simulink model "sampleModel1739_2"  (R2023a)
settings: Solver=VariableStepAuto  StartTime=0.0  StopTime=10.0  RelTol=1e-3
libraries: hdlsllib x4, simulink x1
settings Model: Creator=user1  LastModifiedBy=user1

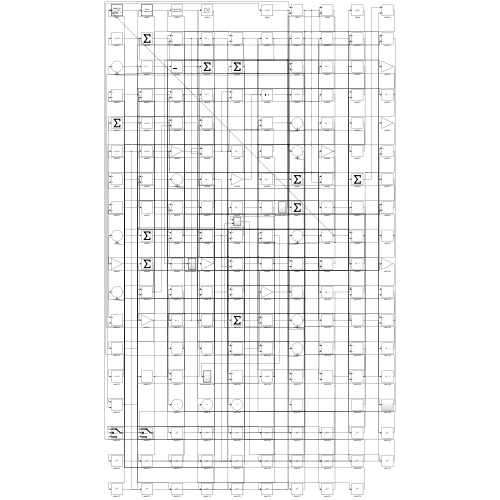
[thumbnail: Simulink's stored preview of the top-level diagram]
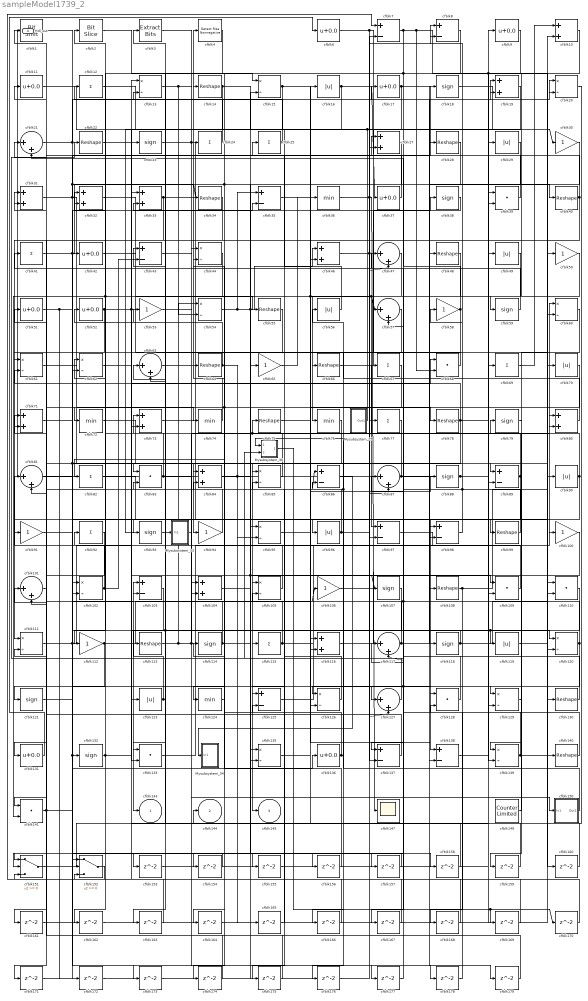
== system sampleModel1739_2 ==
  Mysubsystem_25 : Subsystem  TreatAsAtomicUnit=on  RTWFcnName=Mysubsystem_25
      settings: RTWFcnNameOpts=User specified  RTWFileNameOpts=Use function name
  Mysubsystem_30 : Subsystem  TreatAsAtomicUnit=on  RTWFcnName=Mysubsystem_30
      settings: RTWFcnNameOpts=User specified  RTWFileNameOpts=Use function name
  Mysubsystem_33 : Subsystem  TreatAsAtomicUnit=on  RTWFcnName=Mysubsystem_33
      settings: RTWFcnNameOpts=User specified  RTWFileNameOpts=Use function name
  Mysubsystem_34 : Subsystem  TreatAsAtomicUnit=on  RTWFcnName=Mysubsystem_34
      settings: RTWFcnNameOpts=User specified  RTWFileNameOpts=Use function name
  cfblk1 : hdlsllib/Logic and Bit Operations/Bit Shift  mode=Shift Left Logical  N=0
  cfblk{10,19,27,31..33,46,71,73,80,84,104,116} (13 alike) : Sum  OutDataTypeStr=uint8
  cfblk{30,50,53,58,65,91,94,100,106,112} (10 alike) : Gain  OutDataTypeStr=uint8
  cfblk{21,47,57,63,81,87,101,117,127} (9 alike) : Sum  Inputs=|++  OutDataTypeStr=uint8
  cfblk{13,15,20,44,54,60..62,85,95,102,105,111,120,126,129,135,139} (18 alike) : Product  Inputs=*/  OutDataTypeStr=uint8  RndMeth=Zero  SaturateOnIntegerOverflow=on
  cfblk{7..8,35,43,86,89,97..98,103,125,137..138} (12 alike) : Sum  Inputs=+-  OutDataTypeStr=uint8
  cfblk{18,23,38,59,79,88,93,107,114,118,121,132} (12 alike) : Signum
  cfblk{14,22,28,34,40,48,55,64,66,75,78,99,108,113,130,140} (16 alike) : Reshape
  cfblk{39,68,83,109..110,128,133,141} (8 alike) : DotProduct  OutDataTypeStr=uint8
  cfblk{6,9,11,17,37,42,51..52,131,136} (10 alike) : Bias  Bias=0.0  SaturateOnIntegerOverflow=off
  cfblk{12,24..25,41,67,69,77,82,92,115} (10 alike) : Sum  Inputs=+  OutDataTypeStr=uint8
  cfblk{16,29,49,56,70,90,96,119,123} (9 alike) : Abs  OutDataTypeStr=uint8  SaturateOnIntegerOverflow=off
  cfblk{36,72,74,76,124} (5 alike) : MinMax  OutDataTypeStr=uint8
  cfblk147 : Scope
  cfblk149 : hdlsllib/Sources/Counter Limited  uplimit=7  tsamp=-1
  cfblk150 : Subsystem
      settings: LibrarySourceBlock=|
      | hdlsllib/Ports &
      | Subsystems/Subsystem
  cfblk151 : Switch  OutDataTypeStr=uint8  SaturateOnIntegerOverflow=off  InputSameDT=off
  cfblk152 : Switch  OutDataTypeStr=uint8  SaturateOnIntegerOverflow=off  InputSameDT=off
  cfblk{153..179} (27 alike) : Delay  SampleTime=1
  cfblk2 : hdlsllib/Logic and Bit Operations/Bit Slice  lidx=7  ridx=0
  cfblk3 : simulink/Logic and Bit Operations/Extract Bits  bitsToExtract=Upper half  numBits=8  bitIdxRange=[0 7]  outScalingMode=Preserve fixed-point scaling
      settings: LibrarySourceBlock=|
      | hdlsllib/Logic and Bit
      | Operations/Extract Bits
  cfblk4 : hdlsllib/Logic and Bit Operations/Detect Rise Nonnegative  vinit=0  OutDataTypeStr=uint8
  cfblk143 : Outport  OutDataTypeStr=uint8  VectorParamsAs1DForOutWhenUnconnected=off
  cfblk144 : Outport  Port=2  OutDataTypeStr=uint8  VectorParamsAs1DForOutWhenUnconnected=off
  cfblk145 : Outport  Port=3  OutDataTypeStr=uint8  VectorParamsAs1DForOutWhenUnconnected=off
  Hdl_out : Outport  Port=4  OutDataTypeStr=uint8
  wires:
  cfblk24/1 -> cfblk4/1
  cfblk77/1 -> cfblk94/1
  cfblk34/1 -> cfblk111/1
  cfblk8/1 -> cfblk82/1
  cfblk130/1 -> cfblk92/1
  cfblk85/1 -> cfblk75/1, cfblk43/1
  cfblk140/1 -> cfblk22/1
  cfblk63/1 -> cfblk89/1
  cfblk131/1 -> cfblk6/1
  cfblk65/1 -> cfblk36/1
  cfblk93/1 -> cfblk150/1(In1)
  cfblk79/1 -> cfblk139/1
  cfblk73/1 -> cfblk138/1
  cfblk69/1 -> cfblk10/1
  cfblk36/1 -> cfblk147/1, cfblk138/2
  cfblk21/1 -> cfblk120/1, cfblk17/1
  cfblk33/1 -> cfblk96/1, cfblk102/2
  cfblk66/1 -> cfblk38/1
  cfblk27/1 -> cfblk163/1, cfblk164/1
  cfblk103/1 -> cfblk143/1
  cfblk49/1 -> cfblk97/1, cfblk121/1
  cfblk111/1 -> cfblk23/1, cfblk35/2
  cfblk96/1 -> cfblk71/1, cfblk8/2
  cfblk78/1 -> cfblk145/1, cfblk61/2, cfblk20/2
  cfblk133/1 -> cfblk60/1
  cfblk55/1 -> cfblk61/1
  cfblk108/1 -> cfblk10/2, cfblk168/1
  cfblk70/1 -> cfblk124/1, cfblk101/2
  cfblk31/1 -> cfblk84/1, cfblk27/1
  cfblk37/1 -> cfblk3/1
  cfblk4/1 -> cfblk93/1
  cfblk41/1 -> cfblk140/1, cfblk178/1
  cfblk9/1 -> cfblk72/1, cfblk137/1
  cfblk20/1 -> cfblk144/1
  cfblk115/1 -> cfblk39/1, cfblk21/1
  cfblk151/1 -> cfblk49/1
  cfblk113/1 -> cfblk9/1, cfblk80/1, cfblk54/1
  cfblk87/1 -> cfblk85/1, cfblk179/1
  cfblk106/1 -> cfblk29/1
  cfblk105/1 -> cfblk63/1
  cfblk12/1 -> cfblk98/1
  cfblk47/1 -> cfblk76/1
  cfblk35/1 -> cfblk16/1
  cfblk125/1 -> cfblk50/1
  cfblk141/1 -> cfblk136/1, cfblk31/1
  cfblk124/1 -> cfblk84/2
  cfblk52/1 -> cfblk123/1, cfblk90/1, cfblk81/2
  cfblk123/1 -> cfblk103/1, cfblk153/1
  cfblk71/1 -> cfblk89/2, cfblk156/1
  cfblk116/1 -> cfblk48/1
  cfblk89/1 -> cfblk67/1, cfblk155/1
  cfblk101/1 -> cfblk51/1
  cfblk48/1 -> cfblk115/1
  cfblk6/1 -> cfblk108/1, cfblk127/2
  cfblk149/1 -> cfblk79/1
  cfblk74/1 -> cfblk14/1
  cfblk14/1 -> cfblk63/2, cfblk27/2
  cfblk137/1 -> cfblk101/1
  cfblk17/1 -> cfblk105/1, cfblk40/1
  cfblk2/1 -> cfblk15/1
  cfblk62/1 -> cfblk99/1
  cfblk59/1 -> cfblk47/1
  cfblk15/1 -> cfblk57/1, cfblk78/1, cfblk73/2
  cfblk95/1 -> cfblk88/1
  cfblk138/1 -> cfblk69/1
  cfblk23/1 -> cfblk135/1, cfblk128/1
  cfblk120/1 -> cfblk166/1, cfblk167/1, cfblk64/1
  cfblk42/1 -> cfblk118/1
  cfblk126/1 -> cfblk105/2
  cfblk90/1 -> cfblk151/1, cfblk53/1
  cfblk104/1 -> cfblk65/1
  cfblk29/1 -> cfblk42/1
  cfblk97/1 -> cfblk100/1
  cfblk94/1 -> cfblk13/2
  cfblk150/1(Out1) -> Mysubsystem_30/1(In1), cfblk86/1
  cfblk98/1 -> cfblk58/1
  cfblk54/1 -> cfblk46/1, cfblk126/2, cfblk35/1
  cfblk16/1 -> cfblk37/1, cfblk174/1
  cfblk13/1 -> cfblk44/1, cfblk54/2
  cfblk81/1 -> cfblk98/2
  cfblk92/1 -> cfblk131/1
  cfblk91/1 -> cfblk152/1
  cfblk32/1 -> cfblk55/1
  cfblk114/1 -> cfblk71/2, cfblk28/1
  cfblk10/1 -> cfblk59/1
  cfblk152/1 -> cfblk7/1
  cfblk109/1 -> cfblk2/1
  cfblk83/1 -> cfblk52/1, cfblk80/2
  cfblk56/1 -> cfblk25/1
  cfblk132/1 -> cfblk68/1, cfblk32/2, cfblk162/1
  cfblk11/1 -> cfblk77/1
  cfblk40/1 -> cfblk18/1, cfblk171/1
  cfblk7/1 -> cfblk70/1, cfblk129/2, cfblk68/2, cfblk117/2
  cfblk82/1 -> cfblk110/1
  cfblk110/1 -> cfblk133/1, cfblk133/2, cfblk119/1
  cfblk50/1 -> cfblk112/1, cfblk141/2
  cfblk64/1 -> cfblk32/1, cfblk165/1
  cfblk102/1 -> cfblk81/1, cfblk43/2
  cfblk57/1 -> cfblk83/1
  cfblk75/1 -> cfblk116/2
  cfblk99/1 -> cfblk41/1, cfblk8/1
  cfblk18/1 -> cfblk130/1
  cfblk68/1 -> cfblk66/1
  cfblk60/1 -> cfblk129/1
  cfblk80/1 -> cfblk56/1
  cfblk58/1 -> cfblk126/1, cfblk21/2
  cfblk46/1 -> cfblk47/2, cfblk19/2
  cfblk51/1 -> cfblk132/1, cfblk173/1, cfblk172/1
  cfblk39/1 -> cfblk11/1
  cfblk38/1 -> cfblk33/2
  cfblk139/1 -> cfblk106/1, cfblk73/1, cfblk110/2
  cfblk25/1 -> cfblk12/1, cfblk175/1
  cfblk30/1 -> cfblk135/2
  cfblk72/1 -> cfblk104/1
  cfblk88/1 -> cfblk139/2, Hdl_out/1
  cfblk43/1 -> cfblk104/2
  cfblk44/1 -> cfblk91/1
  cfblk100/1 -> cfblk125/1
  cfblk121/1 -> cfblk103/2
  cfblk117/1 -> cfblk62/1, cfblk20/1
  cfblk61/1 -> cfblk74/1
  cfblk128/1 -> cfblk87/1
  cfblk22/1 -> cfblk109/1
  cfblk112/1 -> cfblk141/1, cfblk46/2
  cfblk1/1 -> cfblk34/1, cfblk127/1
  cfblk3/1 -> cfblk24/1
  cfblk84/1 -> cfblk107/1, cfblk158/1, cfblk95/2
  cfblk118/1 -> cfblk60/2, cfblk113/1
  cfblk136/1 -> cfblk114/1, cfblk86/2
  cfblk135/1 -> cfblk19/1
  cfblk153/1 -> cfblk109/2
  cfblk67/1 -> cfblk154/1
  cfblk154/1 -> cfblk152/2
  cfblk155/1 -> cfblk87/2
  cfblk156/1 -> cfblk44/2
  cfblk28/1 -> cfblk157/1
  cfblk157/1 -> cfblk151/2
  cfblk158/1 -> cfblk83/2
  cfblk129/1 -> cfblk159/1
  cfblk159/1 -> cfblk13/1
  cfblk119/1 -> cfblk160/1
  cfblk160/1 -> cfblk116/1
  cfblk76/1 -> cfblk161/1
  cfblk161/1 -> cfblk39/2
  cfblk162/1 -> cfblk15/2
  cfblk163/1 -> cfblk33/1
  cfblk164/1 -> cfblk120/2
  cfblk165/1 -> cfblk85/2
  cfblk166/1 -> cfblk152/3
  cfblk167/1 -> cfblk125/2
  cfblk168/1 -> cfblk102/1
  cfblk169/1 -> cfblk57/2
  cfblk170/1 -> cfblk151/3
  cfblk171/1 -> cfblk62/2
  cfblk172/1 -> cfblk95/1
  cfblk173/1 -> cfblk7/2
  cfblk174/1 -> cfblk31/2
  cfblk175/1 -> cfblk111/2
  cfblk107/1 -> cfblk176/1
  cfblk176/1 -> cfblk97/2
  cfblk53/1 -> cfblk177/1
  cfblk177/1 -> cfblk117/1
  cfblk178/1 -> cfblk128/2
  cfblk179/1 -> cfblk1/1
  Mysubsystem_25/1(Out1) -> cfblk137/2, cfblk30/1
  Mysubsystem_30/1(Out1) -> cfblk169/1, cfblk170/1
  cfblk127/1 -> Mysubsystem_30/2(In2)
  cfblk19/1 -> Mysubsystem_33/1(In1)
  cfblk86/1 -> Mysubsystem_34/1(In1)

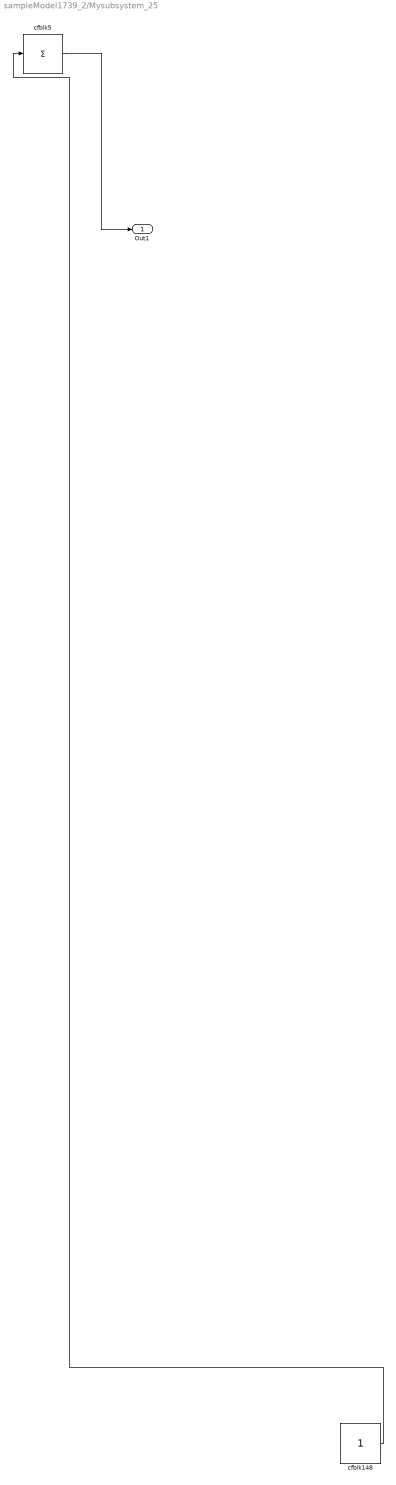
== system sampleModel1739_2/Mysubsystem_25 ==
  cfblk148 : Constant  SampleTime=-1
  cfblk5 : Sum  Inputs=+
  Out1 : Outport
  wires:
  cfblk148/1 -> cfblk5/1
  cfblk5/1 -> Out1/1

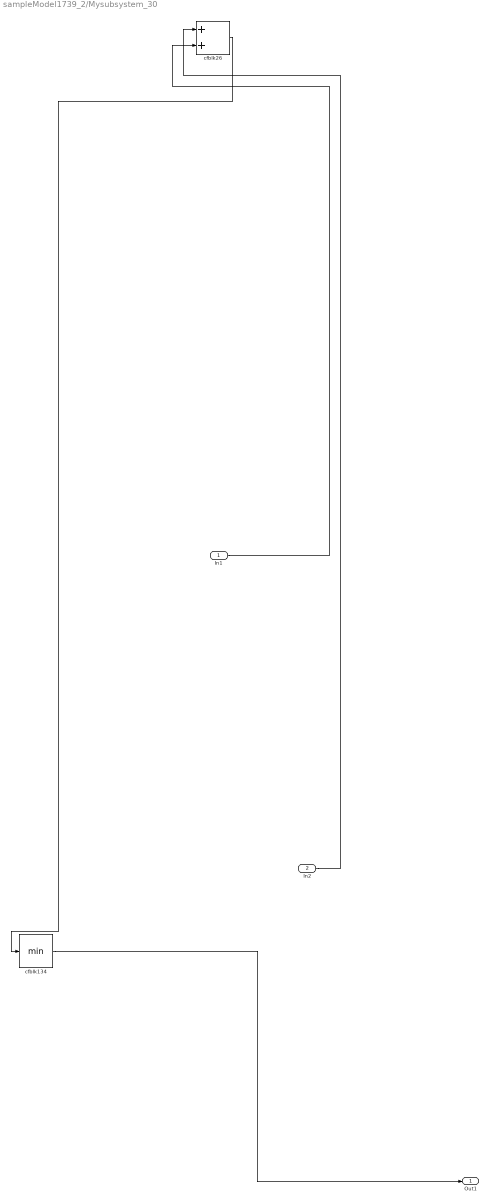
== system sampleModel1739_2/Mysubsystem_30 ==
  In1 : Inport
  In2 : Inport  Port=2
  cfblk134 : MinMax
  cfblk26 : Sum
  Out1 : Outport
  wires:
  cfblk26/1 -> cfblk134/1
  cfblk134/1 -> Out1/1
  In2/1 -> cfblk26/1
  In1/1 -> cfblk26/2

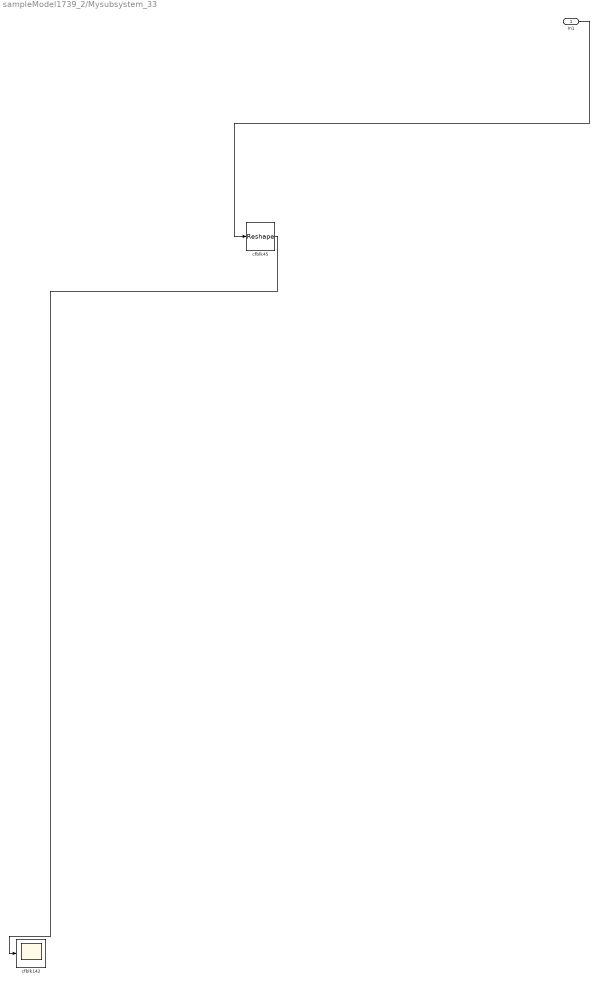
== system sampleModel1739_2/Mysubsystem_33 ==
  In1 : Inport
  cfblk142 : Scope
  cfblk45 : Reshape
  wires:
  cfblk45/1 -> cfblk142/1
  In1/1 -> cfblk45/1

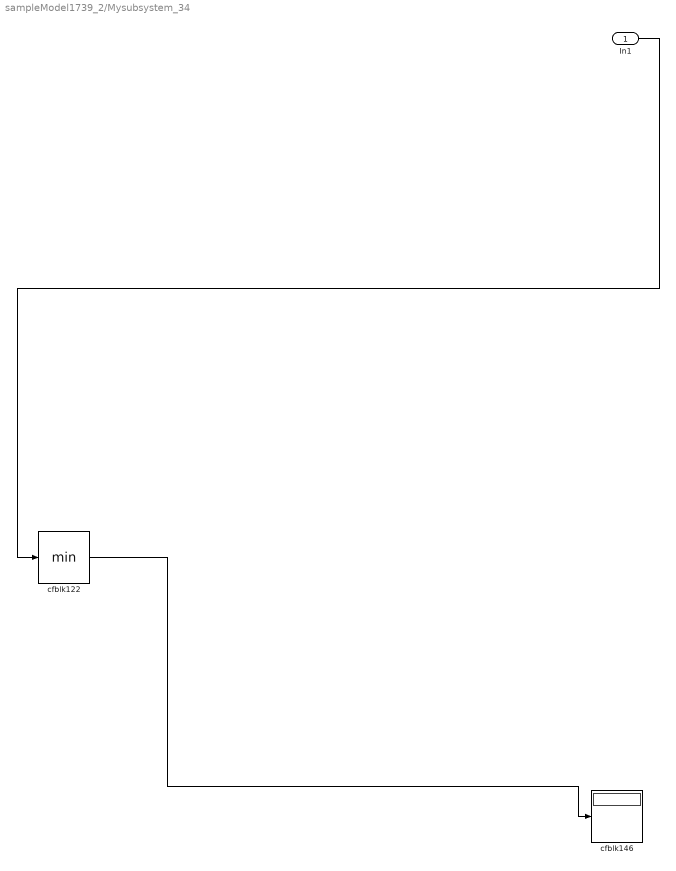
== system sampleModel1739_2/Mysubsystem_34 ==
  In1 : Inport
  cfblk122 : MinMax
  cfblk146 : Display
  wires:
  cfblk122/1 -> cfblk146/1
  In1/1 -> cfblk122/1

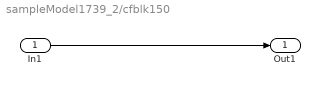
== system sampleModel1739_2/cfblk150 ==
  In1 : Inport
  Out1 : Outport
  wires:
  In1/1 -> Out1/1
